simulink model "fll921"  (R2023a)
settings: Solver=ode45  StartTime=0.0  StopTime=0.12  RelTol=1e-6
model workspace (MAT data in the model file):
  K = 1
libraries: spsIGBTDiodeLib x6, spsabctoAlphaBetaZeroLib x4, spsAlphaBetaZerotoabcLib x2, spsAlphaBetaZerotodq0Lib x2, slpidlib x2, spsSawtoothGeneratorLib x2, cstextras x2, spsThreePhaseSeriesRLCBranchLib x2, spsThreePhaseVIMeasurementLib x2, spsGroundLib x1, spsDCVoltageSourceLib x1, spsSeriesRLCBranchLib x1
settings Model: Creator=Admin  LastModifiedBy=asus
settings SolverCC: ZeroCrossAlgorithm=Adaptive
settings DebuggingCC: IgnoredZcDiagnostic=none  UnconnectedInputMsg=warning  UnconnectedOutputMsg=warning  UnconnectedLineMsg=warning
settings ModelReferenceCC: EnableRefExpFcnMdlSchedulingChecks=on
settings RTWCC: DLArmComputeVersion=19.05

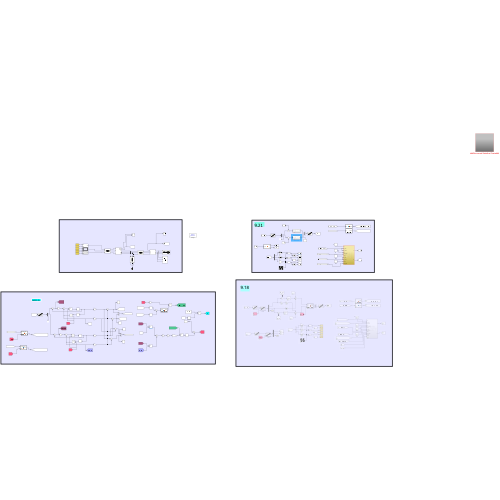
[thumbnail: Simulink's stored preview of the top-level diagram]
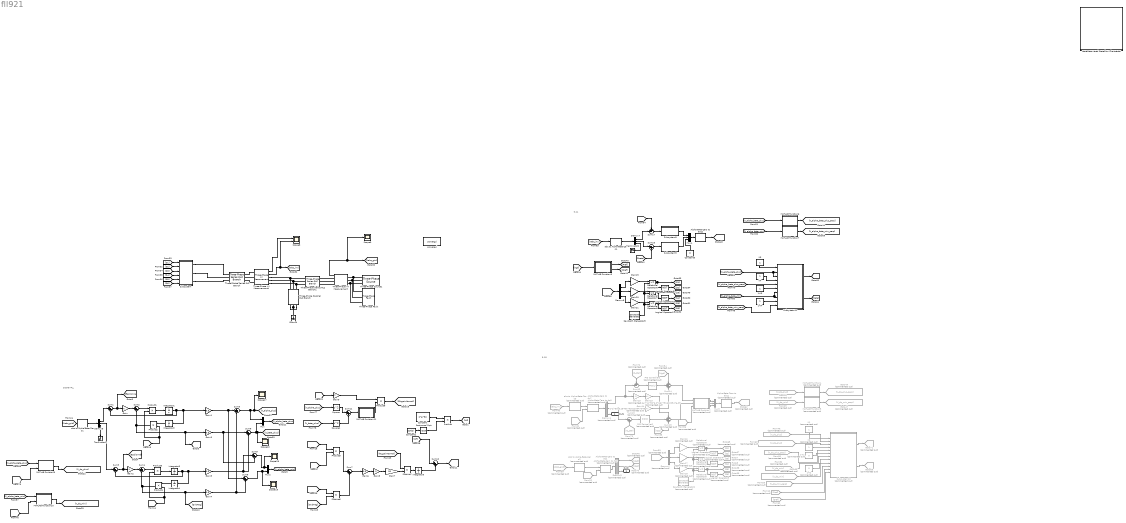
== system fll921 ==
  note: DSOGI-FLL
  note: 9.21
  note: 9.18
  ###Recovered Stateflow Charts### : Subsystem
  1-K1 : Constant  Commented=on  Value=0
  1-K2 : Constant  Commented=on  Value=0
  1-K3 : Constant
  1-K4 : Constant
  Alpha-Beta-Zero to abc1 : spsAlphaBetaZerotoabcLib/Alpha-Beta-Zero to abc  Commented=on
  Alpha-Beta-Zero to abc2 : spsAlphaBetaZerotoabcLib/Alpha-Beta-Zero to abc
  Alpha-Beta-Zero to dq1 : spsAlphaBetaZerotodq0Lib/Alpha-Beta-Zero to dq0  Commented=on  Alignment=90 degrees behind phase A axis
  Alpha-Beta-Zero to dq2 : spsAlphaBetaZerotodq0Lib/Alpha-Beta-Zero to dq0  Commented=on  Alignment=90 degrees behind phase A axis
  Constant : Constant  Value=2*pi*50
  Constant1 : Constant  Value=sqrt(2)
  Constant3 : Constant  Value=0
  Demux3 : Demux  Commented=on  Outputs=3
  Demux4 : Demux  Commented=on  Outputs=3
  Demux5 : Demux  Outputs=3
  Demux6 : Demux  Commented=on  Outputs=3
  Demux7 : Demux  Outputs=3
  Demux8 : Demux  Outputs=3
  From12 : From  Commented=on  GotoTag=Pref
  From20 : From  Commented=on  GotoTag=omega
  From21 : From  Commented=on  GotoTag=omega
  From28 : From  Commented=on  GotoTag=V_dq_plus
  From29 : From  Commented=on  GotoTag=V_dq_min
  From39 : From  Commented=on  GotoTag=Vabc_grid
  From40 : From  Commented=on  GotoTag=Iabc_inv
  From49 : From  Commented=on  GotoTag=V_dq_plus
  From50 : From  Commented=on  GotoTag=V_dq_plus_perp
  From52 : From  Commented=on  GotoTag=V_dq_min
  From53 : From  Commented=on  GotoTag=V_dq_min_perp
  From54 : From  Commented=on  GotoTag=Vgd
  From55 : From  Commented=on  GotoTag=Vgq
  From56 : From  Commented=on  GotoTag=omega
  From59 : From  Commented=on  GotoTag=Vabc_inv
  From62 : From  Commented=on  GotoTag=Qref
  From68 : From  Commented=on  GotoTag=V_dq_plus
  From69 : From  Commented=on  GotoTag=V_dq_min
  From72 : From  Commented=on  GotoTag=Id_star
  From73 : From  Commented=on  GotoTag=Iq_star
  Gain : Gain  Gain=K
  Gain{1,3..6} (5 alike) : Gain  Gain=0.5
  Gain13 : Gain  Commented=on  Gain=2*pi*50*6.254627916220947e-05
  Gain14 : Gain  Commented=on  Gain=2*pi*50*6.254627916220947e-05
  Gain15 : Gain  Commented=on  Gain=-1
  Gain16 : Gain  Commented=on  Gain=2/800
  Gain17 : Gain  Commented=on  Gain=2/800
  Gain18 : Gain  Commented=on  Gain=2/800
  Gain19 : Gain  Gain=2/800
  Gain2 : Gain  Gain=K
  Gain20 : Gain  Gain=2/800
  Gain21 : Gain  Gain=2/800
  Gain7 : Gain  Gain=50
  Gain8 : Gain  Gain=-1
  Gain9 : Gain  Gain=K
  Goto38 : Goto  Commented=on  GotoTag=S5
  Goto39 : Goto  Commented=on  GotoTag=S6
  Goto43 : Goto  Commented=on  GotoTag=V_dq_plus_perp
  Goto46 : Goto  Commented=on  GotoTag=Vgd
  Goto47 : Goto  Commented=on  GotoTag=V_dq_min_perp
  Goto62 : Goto  Commented=on  GotoTag=Vabc_inv
  Goto65 : Goto  Commented=on  GotoTag=S1
  Goto67 : Goto  Commented=on  GotoTag=S2
  Goto68 : Goto  Commented=on  GotoTag=Iq_star
  Goto7 : Goto  Commented=on  GotoTag=S3
  Goto70 : Goto  Commented=on  GotoTag=Vgq
  Goto71 : Goto  Commented=on  GotoTag=Id_star
  Goto8 : Goto  Commented=on  GotoTag=S4
  Ground : spsGroundLib/Ground  LConnTagsString=a
  Integrator{1..5} (5 alike) : Integrator
  "K1 " : Constant  Commented=on
  K2 : Constant  Commented=on
  K3 : Constant
  K4 : Constant
  Logical Operator10 : Logic  Operator=NOT  AllPortsSameDT=off  OutDataTypeStr=boolean
  Logical Operator11 : Logic  Operator=NOT  AllPortsSameDT=off  OutDataTypeStr=boolean
  Logical Operator3 : Logic  Commented=on  Operator=NOT  AllPortsSameDT=off  OutDataTypeStr=boolean
  Logical Operator4 : Logic  Commented=on  Operator=NOT  AllPortsSameDT=off  OutDataTypeStr=boolean
  Logical Operator5 : Logic  Commented=on  Operator=NOT  AllPortsSameDT=off  OutDataTypeStr=boolean
  Logical Operator9 : Logic  Operator=NOT  AllPortsSameDT=off  OutDataTypeStr=boolean
  MATLAB Function10 : MATLAB Function  TreatAsAtomicUnit=on
  MATLAB Function11 : MATLAB Function  TreatAsAtomicUnit=on
  MATLAB Function2 : MATLAB Function  Commented=on  TreatAsAtomicUnit=on
  MATLAB Function3 : MATLAB Function  TreatAsAtomicUnit=on
  MATLAB Function4 : MATLAB Function  Commented=on  TreatAsAtomicUnit=on
  MATLAB Function5 : MATLAB Function  Commented=on  TreatAsAtomicUnit=on
  MATLAB Function6 : MATLAB Function  TreatAsAtomicUnit=on
  MATLAB Function7 : MATLAB Function  TreatAsAtomicUnit=on
  MATLAB Function9 : MATLAB Function  TreatAsAtomicUnit=on
  Mux : Mux  Inputs=2
  Mux2 : Mux  Inputs=2
  Mux3 : Mux  Commented=on  Inputs=3
  Mux4 : Mux  Inputs=3
  PID Controller1 : slpidlib/PID Controller  Commented=on  Controller=PID  Form=Parallel  TimeDomain=Discrete-time  UseExternalTs=off  SampleTime=-1  IntegratorMethod=Forward Euler  FilterMethod=Forward Euler  ControllerParametersSource=internal  P=5  I=1  UseKiTs=off  D=0  N=100  UseFilter=on  TunerSelectOption=Transfer Function Based (PID Tuner App)  InitialConditionSource=internal  InitialConditionForIntegrator=0  InitialConditionForFilter=0  DifferentiatorICPrevScaledInput=0  ExternalReset=none  TrackingMode=off  Kt=1  LimitOutput=off  SatLimitsSource=internal  UpperSaturationLimit=inf  LowerSaturationLimit=-inf  LinearizeAsGain=on  AntiWindupMode=none  Kb=1  LimitIntegrator=off  UpperIntegratorSaturationLimit=inf  LowerIntegratorSaturationLimit=-inf  POutMin=[]  POutMax=[]  IOutMin=[]  IOutMax=[]  DOutMin=[]  DOutMax=[]  NOutMin=[]  NOutMax=[]  SumOutMin=[]  SumOutMax=[]  SaturationOutMin=[]  SaturationOutMax=[]  PParamMin=[]  PParamMax=[]  IParamMin=[]  IParamMax=[]  DParamMin=[]  DParamMax=[]  NParamMin=[]  NParamMax=[]  KbParamMin=[]  KbParamMax=[]  KtParamMin=[]  KtParamMax=[]  KbOutMin=[]  KbOutMax=[]  KtOutMin=[]  KtOutMax=[]  IntegratorOutMin=[]  IntegratorOutMax=[]  FilterOutMin=[]  FilterOutMax=[]  SumI1OutMin=[]  SumI1OutMax=[]  SumI2OutMin=[]  SumI2OutMax=[]  SumI3OutMin=[]  SumI3OutMax=[]  SumI4OutMin=[]  SumI4OutMax=[]  SumDOutMin=[]  SumDOutMax=[]  DifferentiatorOutMin=[]  DifferentiatorOutMax=[]  FilterDiffOutCoefMin=[]  FilterDiffOutCoefMax=[]  ReciprocalOutMin=[]  ReciprocalOutMax=[]  SumDenOutMin=[]  SumDenOutMax=[]  SumNumOutMin=[]  SumNumOutMax=[]  DivideOutMin=[]  DivideOutMax=[]  UdiffTsProdOutMin=[]  UdiffTsProdOutMax=[]  NTsProdOutMin=[]  NTsProdOutMax=[]  UintegralTsProdOutMin=[]  UintegralTsProdOutMax=[]  UngainTsProdOutMin=[]  UngainTsProdOutMax=[]  ClampingZeroOutDataTypeStr=Inherit: Inherit via back propagation  ClampingZeroOutMin=[]  ClampingZeroOutMax=[]  FilterDenConstantOutDataTypeStr=Inherit: Inherit via back propagation  FilterDenConstantOutMin=[]  FilterDenConstantOutMax=[]  PCopyOutDataTypeStr=Inherit: Inherit via back propagation  PCopyOutMin=[]  PCopyOutMax=[]  NCopyOutDataTypeStr=Inherit: Inherit via back propagation  NCopyOutMin=[]  NCopyOutMax=[]  IntegratorContinuousStateAttributes=''  IntegratorStateMustResolveToSignalObject=off  IntegratorRTWStateStorageClass=Auto  FilterContinuousStateAttributes=''  FilterStateMustResolveToSignalObject=off  FilterRTWStateStorageClass=Auto  ParallelPVariant=InternalParameters  IdealPVariant=Disabled  IVariant=InternalParameters  DVariant=InternalParameters  IntegratorVariant=Discrete  SatVariant=Disabled  AWVariant=Passthrough  PCopyVariant=Disabled  TRVariant=Disabled  FdbkBlocksVariant=Forward  IdealPFdbkVariant=Disabled  SatFdbkVariant=Disabled  DerivativeFilterVariant=ForwardEulerFilter  NVariant=InternalParameters  NCopyVariant=Disabled  FilterICVariant=InternalICsFilter  IntegratorICVariant=InternalICs  ExternalResetVariant=Disabled  TRSumVariant=Passthrough  SumFdbkVariant=Disabled  SumVariant=Sum_PID  TsampFilterVariant=InternalTs  TsampNgainVariant=Passthrough  TsampIntegralVariant=Disabled_SignalSpec  ExternalSaturationOutDataTypeStr=Inherit: Same as second input
  PID Controller2 : slpidlib/PID Controller  Commented=on  Controller=PID  Form=Parallel  TimeDomain=Discrete-time  UseExternalTs=off  SampleTime=-1  IntegratorMethod=Forward Euler  FilterMethod=Forward Euler  ControllerParametersSource=internal  P=5  I=1  UseKiTs=off  D=0  N=100  UseFilter=on  TunerSelectOption=Transfer Function Based (PID Tuner App)  InitialConditionSource=internal  InitialConditionForIntegrator=0  InitialConditionForFilter=0  DifferentiatorICPrevScaledInput=0  ExternalReset=none  TrackingMode=off  Kt=1  LimitOutput=off  SatLimitsSource=internal  UpperSaturationLimit=inf  LowerSaturationLimit=-inf  LinearizeAsGain=on  AntiWindupMode=none  Kb=1  LimitIntegrator=off  UpperIntegratorSaturationLimit=inf  LowerIntegratorSaturationLimit=-inf  POutMin=[]  POutMax=[]  IOutMin=[]  IOutMax=[]  DOutMin=[]  DOutMax=[]  NOutMin=[]  NOutMax=[]  SumOutMin=[]  SumOutMax=[]  SaturationOutMin=[]  SaturationOutMax=[]  PParamMin=[]  PParamMax=[]  IParamMin=[]  IParamMax=[]  DParamMin=[]  DParamMax=[]  NParamMin=[]  NParamMax=[]  KbParamMin=[]  KbParamMax=[]  KtParamMin=[]  KtParamMax=[]  KbOutMin=[]  KbOutMax=[]  KtOutMin=[]  KtOutMax=[]  IntegratorOutMin=[]  IntegratorOutMax=[]  FilterOutMin=[]  FilterOutMax=[]  SumI1OutMin=[]  SumI1OutMax=[]  SumI2OutMin=[]  SumI2OutMax=[]  SumI3OutMin=[]  SumI3OutMax=[]  SumI4OutMin=[]  SumI4OutMax=[]  SumDOutMin=[]  SumDOutMax=[]  DifferentiatorOutMin=[]  DifferentiatorOutMax=[]  FilterDiffOutCoefMin=[]  FilterDiffOutCoefMax=[]  ReciprocalOutMin=[]  ReciprocalOutMax=[]  SumDenOutMin=[]  SumDenOutMax=[]  SumNumOutMin=[]  SumNumOutMax=[]  DivideOutMin=[]  DivideOutMax=[]  UdiffTsProdOutMin=[]  UdiffTsProdOutMax=[]  NTsProdOutMin=[]  NTsProdOutMax=[]  UintegralTsProdOutMin=[]  UintegralTsProdOutMax=[]  UngainTsProdOutMin=[]  UngainTsProdOutMax=[]  ClampingZeroOutDataTypeStr=Inherit: Inherit via back propagation  ClampingZeroOutMin=[]  ClampingZeroOutMax=[]  FilterDenConstantOutDataTypeStr=Inherit: Inherit via back propagation  FilterDenConstantOutMin=[]  FilterDenConstantOutMax=[]  PCopyOutDataTypeStr=Inherit: Inherit via back propagation  PCopyOutMin=[]  PCopyOutMax=[]  NCopyOutDataTypeStr=Inherit: Inherit via back propagation  NCopyOutMin=[]  NCopyOutMax=[]  IntegratorContinuousStateAttributes=''  IntegratorStateMustResolveToSignalObject=off  IntegratorRTWStateStorageClass=Auto  FilterContinuousStateAttributes=''  FilterStateMustResolveToSignalObject=off  FilterRTWStateStorageClass=Auto  ParallelPVariant=InternalParameters  IdealPVariant=Disabled  IVariant=InternalParameters  DVariant=InternalParameters  IntegratorVariant=Discrete  SatVariant=Disabled  AWVariant=Passthrough  PCopyVariant=Disabled  TRVariant=Disabled  FdbkBlocksVariant=Forward  IdealPFdbkVariant=Disabled  SatFdbkVariant=Disabled  DerivativeFilterVariant=ForwardEulerFilter  NVariant=InternalParameters  NCopyVariant=Disabled  FilterICVariant=InternalICsFilter  IntegratorICVariant=InternalICs  ExternalResetVariant=Disabled  TRSumVariant=Passthrough  SumFdbkVariant=Disabled  SumVariant=Sum_PID  TsampFilterVariant=InternalTs  TsampNgainVariant=Passthrough  TsampIntegralVariant=Disabled_SignalSpec  ExternalSaturationOutDataTypeStr=Inherit: Same as second input
  Product{,1..8} (9 alike) : Product
  Reciprocal Sqrt : Sqrt  Operator=rSqrt  IntermediateResultsDataTypeStr=double
  Relational Operator3 : RelationalOperator  Commented=on  OutDataTypeStr=boolean  RndMeth=Simplest  InputSameDT=off
  Relational Operator4 : RelationalOperator  Commented=on  OutDataTypeStr=boolean  RndMeth=Simplest  InputSameDT=off
  Relational Operator5 : RelationalOperator  Commented=on  OutDataTypeStr=boolean  RndMeth=Simplest  InputSameDT=off
  Relational Operator6 : RelationalOperator  OutDataTypeStr=boolean  RndMeth=Simplest  InputSameDT=off
  Relational Operator7 : RelationalOperator  OutDataTypeStr=boolean  RndMeth=Simplest  InputSameDT=off
  Relational Operator8 : RelationalOperator  OutDataTypeStr=boolean  RndMeth=Simplest  InputSameDT=off
  Sawtooth Generator2 : spsSawtoothGeneratorLib/Sawtooth Generator  Commented=on  Freq=120e3  Phase=180  Ts=0
  Sawtooth Generator3 : spsSawtoothGeneratorLib/Sawtooth Generator  Freq=120e3  Phase=180  Ts=0
  Scope{9..10,17..19} (5 alike) : Scope
  Scope8 : Scope  NumInputPorts=2
  Square : Math  Operator=square
  Square1 : Math  Operator=square
  Subsystem : Subsystem
  Subsystem10 : Subsystem  Commented=on
  Subsystem11 : Subsystem
  Subsystem8 : Subsystem
  Subsystem9 : Subsystem
  Sum{1..5,9} (6 alike) : Sum  Inputs=|+-
  Sum{6..8,10..11} (5 alike) : Sum  Inputs=|++
  Sum12 : Sum  Commented=on  Inputs=+-|
  Sum13 : Sum  Commented=on  Inputs=|-+
  Sum14 : Sum  Commented=on  Inputs=+++
  Sum15 : Sum  Commented=on  Inputs=+++
  Sum16 : Sum  Inputs=|-+
  Sum17 : Sum  Inputs=+-|
  Terminator1 : Terminator
  Terminator2 : Terminator
  Three-Phase Parallel RLC Branch : spsThreePhaseParallelRLCBranchLib/Three-Phase Parallel RLC Branch  LConnTagsString=A|B|C  RConnTagsString=A|B|C  BranchType=C  Resistance=1  Inductance=1e-3  Capacitance=4.22171e-05  Measurements=None
  Three-Phase Series RLC Branch : spsThreePhaseSeriesRLCBranchLib/Three-Phase Series RLC Branch  LConnTagsString=A|B|C  RConnTagsString=A|B|C  BranchType=L  Resistance=1  Inductance=25.6e-06  Capacitance=1e-6  Measurements=None
  Three-Phase Series RLC Branch1 : spsThreePhaseSeriesRLCBranchLib/Three-Phase Series RLC Branch  LConnTagsString=A|B|C  RConnTagsString=A|B|C  BranchType=L  Resistance=1  Inductance=5e-06  Capacitance=1e-6  Measurements=None
  Three-Phase V-I Measurement : spsThreePhaseVIMeasurementLib/Three-Phase V-I Measurement  VoltageMeasurement=phase-to-ground  SetLabelV=off  LabelV=Vabc  Vpu=on  VpuLL=off  CurrentMeasurement=no  SetLabelI=off  LabelI=Iabc  Ipu=off  Pbase=100e6  Vbase=400  OutputType=Complex  PhasorSimulation=off  PSBequivalent=0
  Three-Phase V-I Measurement4 : spsThreePhaseVIMeasurementLib/Three-Phase V-I Measurement  VoltageMeasurement=phase-to-ground  SetLabelV=off  LabelV=Vabc  Vpu=on  VpuLL=off  CurrentMeasurement=yes  SetLabelI=off  LabelI=Iabc  Ipu=off  Pbase=100e6  Vbase=400  OutputType=Complex  PhasorSimulation=off  PSBequivalent=0
  Three-Phase Fault : spsThreePhaseFaultLib/Three-Phase Fault  InitialStates=0  FaultA=on  FaultB=on  FaultC=off  GroundFault=off  SwitchTimes="[0.08  0.1]"  External=off  SwitchStatus=NaN  FaultResistance=0.001  GroundResistance=0.01  SnubberResistance=1e6  SnubberCapacitance=inf  Measurements=Fault voltages
  Three-Phase Source1 : spsThreePhaseSourceLib/Three-Phase Source  InternalConnection=Yg  VoltagePhases=off  Voltage=400  PhaseAngle=0  Voltage_phases=[25e3 25e3 25e3]/sqrt(3)  PhaseAngles_phases=[0 -120 +120]  Frequency=50  NonIdealSource=on  SpecifyImpedance=off  Resistance=(3e-3*2*pi*50)/10  Inductance=3e-3  ShortCircuitLevel=160e3  BaseVoltage=400/sqrt(3)  XRratio=10  BusType=PQ  Pref=160e3  Qref=50000  Prefabc=[10e3, 10e3, 10e3]  Qrefabc=[0, 0, 0]  Qmin=-inf  Qmax=inf
  abc to Alpha-Beta-Zero1 : spsabctoAlphaBetaZeroLib/abc to Alpha-Beta-Zero
  abc to Alpha-Beta-Zero2 : spsabctoAlphaBetaZeroLib/abc to Alpha-Beta-Zero  Commented=on
  abc to Alpha-Beta-Zero3 : spsabctoAlphaBetaZeroLib/abc to Alpha-Beta-Zero  Commented=on
  abc to Alpha-Beta-Zero4 : spsabctoAlphaBetaZeroLib/abc to Alpha-Beta-Zero
  powergui : spspowerguiLib/powergui  Priority=1  SimulationMode=Discrete  SampleTime=6.024e-05  frequency=60  Iterations=50  frequencyindice=50  Pbase=100e6  ErrMax=1e-4  UnitsV=kV  UnitsW=MW  buscounter=0  FunctionMessages=off  echomessages=off  EnableUseOfTLC=off  CurrentSourceSwitches=off  DisableSnubberDevices=off  DisableRonSwitches=off  DisableVfSwitches=off  DisplayEquations=off  AutomaticDiscreteSolvers=off  SolverType=Tustin/Backward Euler (TBE)  Interpol=off  ExternalGateDelay=off  methode=off  Ts=100  x0status=blocks  SPID=on  SwTol=0  HookPort=off  NonlinearTolerance=1e-4  nMaxIteration=100  ContinueOnMaxIteration=off  RestoreLinks=warning  ResistiveCurrentMeasurement=off  Frange=[0:2:500]  Ylog=off  Xlog=on  ShowGrid=off  save=off  variable=ZData  structure=0  ZoomFFT=off  StartTime=0.0  cycles=1  DisplayStyle=1  fundamental=60  FreqAxis=off  MaxFrequency=1000  frequencyindicesteady=1  RmsSteady=1  display=off
  Out1 : Outport
  Out2 : Outport  Port=2
  wires:
  Reciprocal Sqrt/1 -> Product/2
  Constant/1 -> Product/1
  Constant1/1 -> Reciprocal Sqrt/1
  Product/1 -> [Wf]
  abc to Alpha-Beta-Zero1/1 -> Demux5/1
  Demux5/1 -> Sum1/1
  Sum1/1 -> [EpsilonVa], Gain/1
  Gain/1 -> Sum2/1
  Sum2/1 -> Product1/1
  Product1/1 -> Integrator1/1
  Integrator1/1 -> Sum1/2, Gain1/1, Integrator2/1
  Integrator2/1 -> Product2/1
  [omega] -> Product2/2, Product1/2
  Product2/1 -> [QvaTag], Gain3/1, Sum2/2
  Sum4/1 -> Product3/1
  Gain2/1 -> Sum4/1
  Integrator3/1 -> Sum3/2, Gain5/1, Integrator4/1
  Product3/1 -> Integrator3/1
  [omega] -> Product4/2, Product3/2
  Integrator4/1 -> Product4/1
  Demux5/2 -> Sum3/1
  Sum3/1 -> [EpsilonVb], Gain2/1
  Gain1/1 -> Sum5/1, Sum6/1
  Gain4/1 -> Sum6/2, Sum5/2
  Sum5/1 -> Mux/1, Scope17/1, [V_alpha_plus]
  Sum6/1 -> Scope19/1, Mux2/2
  Gain3/1 -> Sum8/1, Sum9/2
  Gain5/1 -> Sum9/1, Sum8/2
  Sum8/1 -> Scope10/1, [V_beta_plus], Mux/2
  Sum9/1 -> Scope18/1, Mux2/1
  Product4/1 -> Gain4/1, [QvbTag], Sum4/2
  [EpsilonVa] -> Product5/1
  [QvaTag] -> Product5/2
  [EpsilonVb] -> Product6/1
  [QvbTag] -> Product6/2
  Product5/1 -> Sum7/1
  Product6/1 -> Sum7/2
  Sum7/1 -> Gain6/1
  Gain6/1 -> Gain8/1
  Gain8/1 -> Gain7/1
  Integrator5/1 -> Sum10/2
  [Wf] -> Sum10/1
  Sum10/1 -> [omega]
  [V_alpha_plus] -> Square/1
  [V_beta_plus] -> Square1/1
  Square1/1 -> Sum11/2
  Square/1 -> Sum11/1
  [omega] -> Gain9/1
  Gain9/1 -> Product8/1
  Product8/1 -> [FLLgainNormal]
  [FLLgainNormal] -> Product7/1
  [Vabc_grid] -> abc to Alpha-Beta-Zero1/1
  Three-Phase V-I Measurement4/2 -> Scope8/2, [Iabc_inv]
  [S5] -> Subsystem/5(S5)
  [S1] -> Subsystem/1(S1)
  [S4] -> Subsystem/4(S4)
  [S3] -> Subsystem/3(S3)
  [S2] -> Subsystem/2(S2)
  [S6] -> Subsystem/6(S6)
  Three-Phase V-I Measurement4/1 -> Scope8/1
  Three-Phase V-I Measurement/1 -> Scope9/1, [Vabc_grid]
  Subsystem11/1(Out1) -> [Ialpha]
  [V_alpha_beta_plus] -> Subsystem11/3(V_plus1), Subsystem11/2(V_plus)
  K4/1 -> Subsystem11/4(K2)
  [V_alpha_beta_plus_perp] -> Subsystem11/5(plus_perp)
  1-K3/1 -> Subsystem11/6(1-K1)
  K3/1 -> Subsystem11/1(K1)
  Gain19/1 -> Relational Operator6/1
  [V_alpha_beta_min] -> Subsystem11/7(V_min), Subsystem11/8(V_min1)
  Demux7/2 -> Sum16/1
  1-K4/1 -> Subsystem11/9(1-K2)
  Relational Operator7/1 -> Logical Operator10/1, [S3]
  Subsystem9/1(Out1) -> Mux4/2
  Subsystem10/2(Out2) -> Goto68/1
  Subsystem10/1(Out1) -> Goto71/1
  Gain13/1 -> Sum15/1
  Demux3/2 -> Goto70/1
  From52/1 -> Subsystem10/7(V_min)
  Demux6/2 -> Gain17/1
  1-K2/1 -> Subsystem10/9(1-K2)
  From49/1 -> Subsystem10/2(V_plus)
  From39/1 -> abc to Alpha-Beta-Zero2/1
  Logical Operator4/1 -> Goto8/1
  "K1 "/1 -> Subsystem10/1(K1)
  1-K1/1 -> Subsystem10/6(1-K1)
  Demux7/1 -> Sum17/2
  Gain14/1 -> Sum14/3
  Sum17/1 -> Subsystem8/1(In1)
  Logical Operator10/1 -> [S4]
  MATLAB Function4/1(V_perp) -> Goto43/1
  K2/1 -> Subsystem10/4(K2)
  Sum12/1 -> PID Controller1/1
  From68/1 -> Subsystem10/3(V_plus1)
  Subsystem11/2(Out2) -> [Ibeta]
  abc to Alpha-Beta-Zero4/1 -> Demux7/1
  Logical Operator3/1 -> Goto67/1
  Subsystem8/1(Out1) -> Mux4/1
  Demux8/1 -> Gain19/1
  From59/1 -> Demux6/1
  [Vabc_inv] -> Demux8/1
  Sawtooth Generator3/1 -> Relational Operator6/2, Relational Operator7/2, Relational Operator8/2
  Gain17/1 -> Relational Operator4/1
  Logical Operator9/1 -> [S2]
  Sum16/1 -> Subsystem9/1(In1)
  From53/1 -> Subsystem10/10(min_perp)
  Relational Operator3/1 -> Goto65/1, Logical Operator3/1
  [Ibeta] -> Sum16/2
  MATLAB Function5/1(V_perp) -> Goto47/1
  From56/1 -> MATLAB Function2/3(theta)
  Logical Operator11/1 -> [S6]
  Alpha-Beta-Zero to dq2/1 -> Demux4/1
  Gain15/1 -> Gain13/1
  Demux8/3 -> Gain21/1
  Relational Operator8/1 -> [S5], Logical Operator11/1
  Mux4/1 -> Alpha-Beta-Zero to abc2/1
  Gain20/1 -> Relational Operator7/1
  Logical Operator5/1 -> Goto39/1
  [Iabc_inv] -> abc to Alpha-Beta-Zero4/1
  From72/1 -> Sum12/1
  From54/1 -> Sum14/1
  PID Controller1/1 -> Sum14/2
  From40/1 -> abc to Alpha-Beta-Zero3/1
  Sum13/1 -> PID Controller2/1
  Alpha-Beta-Zero to dq1/1 -> Demux3/1
  Mux3/1 -> Alpha-Beta-Zero to abc1/1
  Demux4/3 -> Out1/1
  Alpha-Beta-Zero to abc2/1 -> [Vabc_inv]
  Gain18/1 -> Relational Operator5/1
  abc to Alpha-Beta-Zero2/1 -> Alpha-Beta-Zero to dq1/1
  Demux4/2 -> Sum13/1, Gain14/1
  From20/1 -> Alpha-Beta-Zero to dq1/2
  From21/1 -> Alpha-Beta-Zero to dq2/2
  Demux6/3 -> Gain18/1
  Relational Operator4/1 -> Logical Operator4/1, Goto7/1
  Demux3/1 -> Goto46/1
  Alpha-Beta-Zero to abc1/1 -> Goto62/1
  abc to Alpha-Beta-Zero3/1 -> Alpha-Beta-Zero to dq2/1
  PID Controller2/1 -> Sum15/2
  Gain16/1 -> Relational Operator3/1
  MATLAB Function6/1(V_perp) -> [V_alpha_beta_plus_perp]
  [Ialpha] -> Sum17/1
  From50/1 -> Subsystem10/5(plus_perp)
  MATLAB Function7/1(V_perp) -> [V_alpha_beta_min_perp]
  Demux3/3 -> Out2/1
  From55/1 -> Sum15/3
  Demux4/1 -> Gain15/1, Sum12/2
  Relational Operator6/1 -> [S1], Logical Operator9/1
  Sawtooth Generator2/1 -> Relational Operator3/2, Relational Operator4/2, Relational Operator5/2
  Relational Operator5/1 -> Goto38/1, Logical Operator5/1
  Gain21/1 -> Relational Operator8/1
  [V_alpha_beta_min_perp] -> Subsystem11/10(min_perp)
  Demux8/2 -> Gain20/1
  Demux6/1 -> Gain16/1
  From73/1 -> Sum13/2
  From69/1 -> Subsystem10/8(V_min1)
  Mux/1 -> [V_alpha_beta_plus]
  Mux2/1 -> [V_alpha_beta_min]
  From29/1 -> MATLAB Function5/1(V)
  From28/1 -> MATLAB Function4/1(V)
  [V_alpha_beta_plus] -> MATLAB Function6/1(V)
  [V_alpha_beta_min] -> MATLAB Function7/1(V)
  From12/1 -> Subsystem10/11(Pref)
  From62/1 -> Subsystem10/12(Qref1)
  MATLAB Function2/2(V_beta) -> Mux3/2
  MATLAB Function2/1(V_alpha) -> Mux3/1
  MATLAB Function2/3(V_zero) -> Mux3/3
  Sum15/1 -> MATLAB Function2/2(V_q)
  Sum14/1 -> MATLAB Function2/1(V_d)
  [omega] -> MATLAB Function9/2(theta)
  [V_alpha_beta_plus] -> MATLAB Function9/1(V_alpha_beta)
  MATLAB Function9/1(V_dq) -> [V_dq_plus]
  [V_alpha_beta_min] -> MATLAB Function10/1(V_alpha_beta)
  [omega] -> MATLAB Function10/2(theta)
  MATLAB Function10/1(V_dq) -> [V_dq_min]
  Demux5/3 -> Terminator1/1
  Gain7/1 -> Product7/2
  Product7/1 -> Integrator5/1
  Sum11/1 -> MATLAB Function11/1(input)
  MATLAB Function11/1(result) -> Product8/2
  Demux7/3 -> Terminator2/1
  Constant3/1 -> Mux4/3
  [Vgd] -> MATLAB Function3/1(V_pu)
  MATLAB Function3/1(P) -> [Pref]
  MATLAB Function3/2(Q) -> [Qref]
  connections:
  Three-Phase Parallel RLC Branch/RConn2 -- Ground/LConn1 -- Three-Phase Parallel RLC Branch/RConn3 -- Three-Phase Parallel RLC Branch/RConn1
  Three-Phase V-I Measurement4/RConn2 -- Three-Phase Series RLC Branch1/LConn2 -- Three-Phase Parallel RLC Branch/LConn2
  Three-Phase V-I Measurement4/RConn1 -- Three-Phase Series RLC Branch1/LConn1 -- Three-Phase Parallel RLC Branch/LConn1
  Three-Phase V-I Measurement4/RConn3 -- Three-Phase Series RLC Branch1/LConn3 -- Three-Phase Parallel RLC Branch/LConn3
  Subsystem/RConn2 -- Three-Phase Series RLC Branch/LConn2
  Subsystem/RConn3 -- Three-Phase Series RLC Branch/LConn3
  Three-Phase V-I Measurement4/LConn1 -- Three-Phase Series RLC Branch/RConn1
  Three-Phase V-I Measurement4/LConn3 -- Three-Phase Series RLC Branch/RConn3
  Three-Phase V-I Measurement4/LConn2 -- Three-Phase Series RLC Branch/RConn2
  Subsystem/RConn1 -- Three-Phase Series RLC Branch/LConn1
  Three-Phase Source1/RConn1 -- Three-Phase Fault/LConn1 -- Three-Phase V-I Measurement/LConn1
  Three-Phase Source1/RConn2 -- Three-Phase Fault/LConn2 -- Three-Phase V-I Measurement/LConn2
  Three-Phase Source1/RConn3 -- Three-Phase Fault/LConn3 -- Three-Phase V-I Measurement/LConn3
  Three-Phase V-I Measurement/RConn1 -- Three-Phase Series RLC Branch1/RConn1
  Three-Phase V-I Measurement/RConn2 -- Three-Phase Series RLC Branch1/RConn2
  Three-Phase V-I Measurement/RConn3 -- Three-Phase Series RLC Branch1/RConn3

== system fll921/###Recovered Stateflow Charts### ==

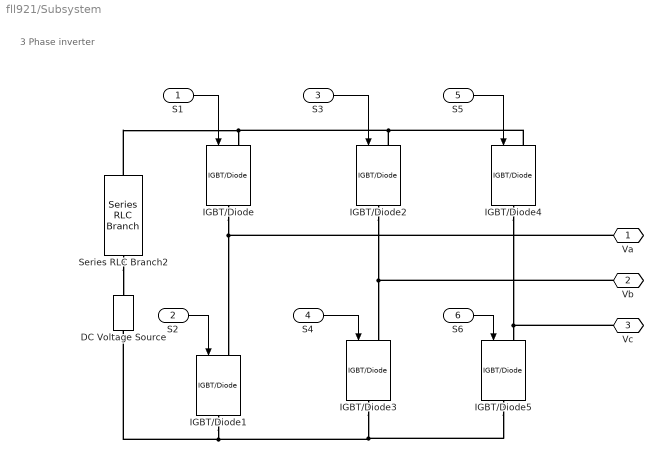
== system fll921/Subsystem ==
  note: 3 Phase inverter
  S1 : Inport
  S2 : Inport  Port=2
  S3 : Inport  Port=3
  S4 : Inport  Port=4
  S5 : Inport  Port=5
  S6 : Inport  Port=6
  DC Voltage Source : spsDCVoltageSourceLib/DC Voltage Source  Amplitude=800  Measurements=None
  IGBT/Diode{,1..5} (6 alike) : spsIGBTDiodeLib/IGBT//Diode  Ron=0.01  Rs=10  Cs=0.1e-6  Measurements=off
  Series RLC Branch2 : spsSeriesRLCBranchLib/Series RLC Branch  LConnTagsString=__new0  RConnTagsString=__new0  BranchType=R  Resistance=0.01  Inductance=1e-3  SetiL0=off  InitialCurrent=0  Capacitance=1e-6  Setx0=off  InitialVoltage=0  Measurements=None
  Va : PMIOPort  Side=Right
  Vb : PMIOPort  Port=2  Side=Right
  Vc : PMIOPort  Port=3  Side=Right
  wires:
  S1/1 -> IGBT/Diode/1
  S2/1 -> IGBT/Diode1/1
  S4/1 -> IGBT/Diode3/1
  S5/1 -> IGBT/Diode4/1
  S3/1 -> IGBT/Diode2/1
  S6/1 -> IGBT/Diode5/1
  connections:
  IGBT/Diode2/RConn1 -- Vb/RConn1 -- IGBT/Diode3/LConn1
  IGBT/Diode/RConn1 -- Va/RConn1 -- IGBT/Diode1/LConn1
  IGBT/Diode2/LConn1 -- Series RLC Branch2/RConn1 -- IGBT/Diode/LConn1 -- IGBT/Diode4/LConn1
  IGBT/Diode3/RConn1 -- IGBT/Diode1/RConn1 -- DC Voltage Source/LConn1 -- IGBT/Diode5/RConn1
  IGBT/Diode4/RConn1 -- Vc/RConn1 -- IGBT/Diode5/LConn1
  Series RLC Branch2/LConn1 -- DC Voltage Source/RConn1

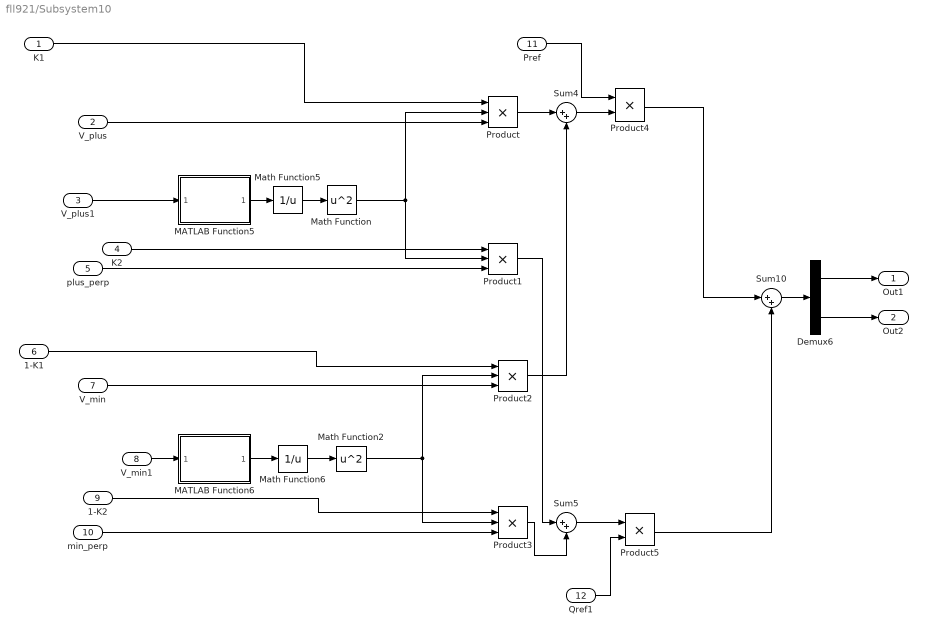
== system fll921/Subsystem10 ==
  K1 : Inport
  V_plus : Inport  Port=2
  V_plus1 : Inport  Port=3
  K2 : Inport  Port=4
  plus_perp : Inport  Port=5
  1-K1 : Inport  Port=6
  V_min : Inport  Port=7
  V_min1 : Inport  Port=8
  1-K2 : Inport  Port=9
  min_perp : Inport  Port=10
  Pref : Inport  Port=11
  Qref1 : Inport  Port=12
  Demux6 : Demux  Outputs=2
  MATLAB Function5 : MATLAB Function  TreatAsAtomicUnit=on
  MATLAB Function6 : MATLAB Function  TreatAsAtomicUnit=on
  Math Function : Math  Operator=square
  Math Function2 : Math  Operator=square
  Math Function5 : Math  Operator=reciprocal
  Math Function6 : Math  Operator=reciprocal
  Product{,1..3} (4 alike) : Product  Inputs=3
  Product4 : Product
  Product5 : Product
  Sum10 : Sum  Inputs=|++
  Sum4 : Sum  Inputs=|++
  Sum5 : Sum  Inputs=|++
  Out1 : Outport
  Out2 : Outport  Port=2
  wires:
  MATLAB Function5/1(v_norm_squared) -> Math Function5/1
  Product3/1 -> Sum5/2
  Math Function6/1 -> Math Function2/1
  Math Function2/1 -> Product2/2, Product3/2
  min_perp/1 -> Product3/3
  Math Function/1 -> Product1/2, Product/2
  Sum5/1 -> Product5/1
  Sum4/1 -> Product4/2
  Product/1 -> Sum4/1
  Product5/1 -> Sum10/2
  K2/1 -> Product1/1
  Demux6/2 -> Out2/1
  1-K1/1 -> Product2/1
  Product4/1 -> Sum10/1
  MATLAB Function6/1(v_norm_squared) -> Math Function6/1
  V_min/1 -> Product2/3
  Product1/1 -> Sum5/1
  Math Function5/1 -> Math Function/1
  Product2/1 -> Sum4/2
  V_min1/1 -> MATLAB Function6/1(V_alpha_beta)
  V_plus1/1 -> MATLAB Function5/1(V_alpha_beta)
  Sum10/1 -> Demux6/1
  Qref1/1 -> Product5/2
  V_plus/1 -> Product/3
  plus_perp/1 -> Product1/3
  1-K2/1 -> Product3/1
  K1/1 -> Product/1
  Demux6/1 -> Out1/1
  Pref/1 -> Product4/1

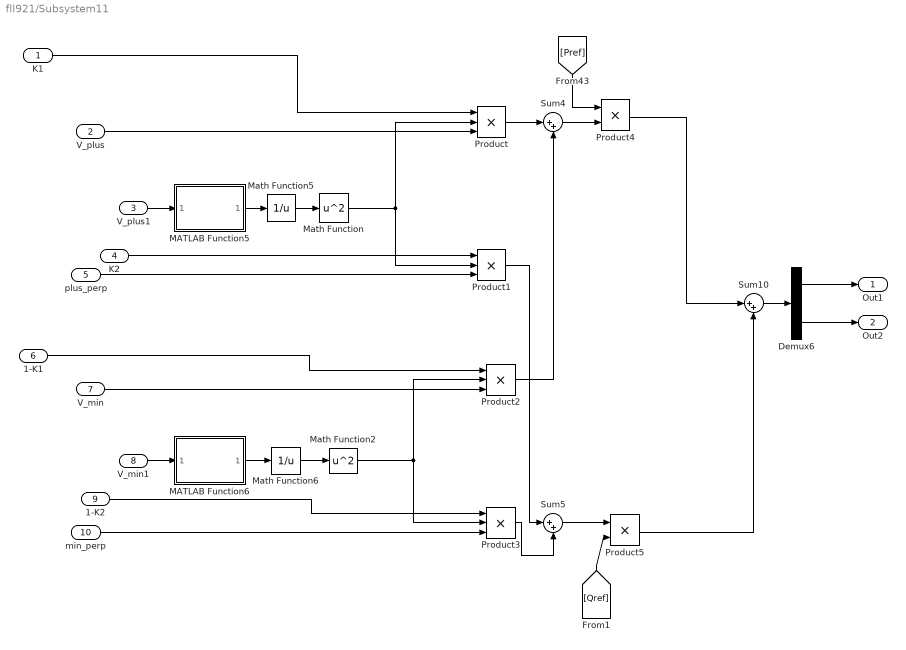
== system fll921/Subsystem11 ==
  K1 : Inport
  V_plus : Inport  Port=2
  V_plus1 : Inport  Port=3
  K2 : Inport  Port=4
  plus_perp : Inport  Port=5
  1-K1 : Inport  Port=6
  V_min : Inport  Port=7
  V_min1 : Inport  Port=8
  1-K2 : Inport  Port=9
  min_perp : Inport  Port=10
  Demux6 : Demux  Outputs=2
  MATLAB Function5 : MATLAB Function  TreatAsAtomicUnit=on
  MATLAB Function6 : MATLAB Function  TreatAsAtomicUnit=on
  Math Function : Math  Operator=square
  Math Function2 : Math  Operator=square
  Math Function5 : Math  Operator=reciprocal
  Math Function6 : Math  Operator=reciprocal
  Product{,1..3} (4 alike) : Product  Inputs=3
  Product4 : Product
  Product5 : Product
  Sum10 : Sum  Inputs=|++
  Sum4 : Sum  Inputs=|++
  Sum5 : Sum  Inputs=|++
  Out1 : Outport
  Out2 : Outport  Port=2
  wires:
  MATLAB Function5/1(v_norm_squared) -> Math Function5/1
  Product3/1 -> Sum5/2
  Math Function6/1 -> Math Function2/1
  Math Function2/1 -> Product2/2, Product3/2
  min_perp/1 -> Product3/3
  Math Function/1 -> Product1/2, Product/2
  Sum5/1 -> Product5/1
  Sum4/1 -> Product4/2
  Product/1 -> Sum4/1
  Product5/1 -> Sum10/2
  K2/1 -> Product1/1
  Demux6/2 -> Out2/1
  1-K1/1 -> Product2/1
  Product4/1 -> Sum10/1
  MATLAB Function6/1(v_norm_squared) -> Math Function6/1
  V_min/1 -> Product2/3
  Product1/1 -> Sum5/1
  Math Function5/1 -> Math Function/1
  Product2/1 -> Sum4/2
  V_min1/1 -> MATLAB Function6/1(V_alpha_beta)
  V_plus1/1 -> MATLAB Function5/1(V_alpha_beta)
  Sum10/1 -> Demux6/1
  [Qref] -> Product5/2
  [Pref] -> Product4/1
  V_plus/1 -> Product/3
  plus_perp/1 -> Product1/3
  1-K2/1 -> Product3/1
  K1/1 -> Product/1
  Demux6/1 -> Out1/1

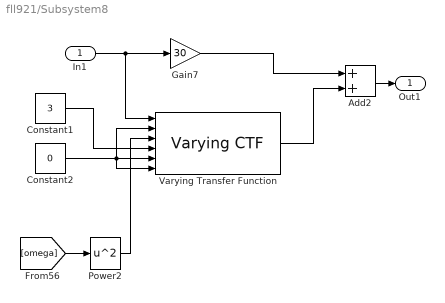
== system fll921/Subsystem8 ==
  In1 : Inport
  Add2 : Sum
  Constant1 : Constant  Value=3
  Constant2 : Constant  Value=0
  Gain7 : Gain  Gain=30
  Power2 : Math  Operator=square
  Varying Transfer Function : cstextras/Varying CTF  N=2
  Out1 : Outport
  wires:
  In1/1 -> Varying Transfer Function/1, Gain7/1
  Gain7/1 -> Add2/1
  Constant1/1 -> Varying Transfer Function/4
  Varying Transfer Function/1 -> Add2/2
  Add2/1 -> Out1/1
  [omega] -> Power2/1
  Constant2/1 -> Varying Transfer Function/2, Varying Transfer Function/6, Varying Transfer Function/5
  Power2/1 -> Varying Transfer Function/3

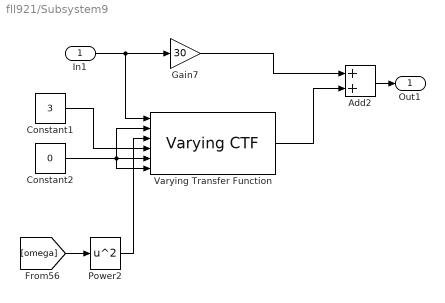
== system fll921/Subsystem9 ==
  In1 : Inport
  Add2 : Sum
  Constant1 : Constant  Value=3
  Constant2 : Constant  Value=0
  Gain7 : Gain  Gain=30
  Power2 : Math  Operator=square
  Varying Transfer Function : cstextras/Varying CTF  N=2
  Out1 : Outport
  wires:
  In1/1 -> Varying Transfer Function/1, Gain7/1
  Gain7/1 -> Add2/1
  Constant1/1 -> Varying Transfer Function/4
  Varying Transfer Function/1 -> Add2/2
  Add2/1 -> Out1/1
  Power2/1 -> Varying Transfer Function/3
  [omega] -> Power2/1
  Constant2/1 -> Varying Transfer Function/5, Varying Transfer Function/6, Varying Transfer Function/2

== matlab function fll921/Subsystem10/MATLAB Function6 ==
  data: V_alpha_beta input; v_norm_squared output
function v_norm_squared = calculateNormSquared(V_alpha_beta)
    v_norm_squared = V_alpha_beta(1)^2 + V_alpha_beta(2)^2;
    if v_norm_squared == 0
        v_norm_squared = NaN;
    end
end

== matlab function fll921/MATLAB Function2 ==
  data: V_d input; V_alpha output; V_q input; theta input; V_beta output; V_zero output
function [V_alpha, V_beta, V_zero] = dq_to_alpha_beta_zero(V_d, V_q, theta)
    % dq_to_alpha_beta_zero: Converts V_d, V_q to V_alpha, V_beta, and V_zero
    %
    % Inputs:
    %   V_d    - Direct-axis voltage component
    %   V_q    - Quadrature-axis voltage component
    %   theta  - Angle of the rotating frame (in radians)
    %
    % Outputs:
    %   V_alpha - Alpha-axis (stationary) voltage component
    %   V_beta  - Beta-axis (stationary) voltage component
    %   V_zero  - Zero-sequence voltage component (typically zero for balanced systems)

    % Compute V_alpha and V_beta using the inverse Park transformation
    V_alpha = V_d * cos(theta) - V_q * sin(theta);
    V_beta  = V_d * sin(theta) + V_q * cos(theta);

    % Compute V_zero (zero-sequence component)
    V_zero = 0;  % Set to zero if there's no zero-sequence component in the system
end

== matlab function fll921/Subsystem11/MATLAB Function5 ==
  data: V_alpha_beta input; v_norm_squared output
function v_norm_squared = calculateNormSquared(V_alpha_beta)
    v_norm_squared = V_alpha_beta(1)^2 + V_alpha_beta(2)^2;
end

== matlab function fll921/Subsystem11/MATLAB Function6 ==
  data: V_alpha_beta input; v_norm_squared output
function v_norm_squared = calculateNormSquared(V_alpha_beta)
    v_norm_squared = V_alpha_beta(1)^2 + V_alpha_beta(2)^2;
end

== matlab function fll921/MATLAB Function9 ==
  data: V_alpha_beta input; V_dq output; theta input
function V_dq = alphaBetaToDQ(V_alpha_beta, theta)
    % V_alpha_beta הוא וקטור דו-ממדי בגודל 2 המכיל את רכיבי האלפא-בטא
    % theta היא הזווית להמרה לתצורת d-q
    
    % חלץ את רכיבי האלפא והבטא
    V_alpha = V_alpha_beta(1);
    V_beta = V_alpha_beta(2);
    
    % בצע את טרנספורמציית ה-Park לתצורת d-q
    V_d = V_alpha * cos(theta) + V_beta * sin(theta);
    V_q = -V_alpha * sin(theta) + V_beta * cos(theta);
    
    % החזר את הווקטור d-q בגודל 2
    V_dq = [V_d; V_q];
end

== matlab function fll921/MATLAB Function10 ==
  data: V_alpha_beta input; V_dq output; theta input
function V_dq = alphaBetaToDQ(V_alpha_beta, theta)
    % V_alpha_beta הוא וקטור דו-ממדי בגודל 2 המכיל את רכיבי האלפא-בטא
    % theta היא הזווית להמרה לתצורת d-q
    
    % חלץ את רכיבי האלפא והבטא
    V_alpha = V_alpha_beta(1);
    V_beta = V_alpha_beta(2);
    
    % בצע את טרנספורמציית ה-Park לתצורת d-q
    V_d = V_alpha * cos(theta) + V_beta * sin(theta);
    V_q = -V_alpha * sin(theta) + V_beta * cos(theta);
    
    % החזר את הווקטור d-q בגודל 2
    V_dq = [V_d; V_q];
end

== matlab function fll921/MATLAB Function11 ==
  data: input input; result output
function result = safeReciprocal(input)
    % Define a small epsilon to avoid division by zero
    epsilon = 1e-6;

    % Calculate the reciprocal, adding epsilon if input is zero or very small
    if abs(input) < epsilon
        result = 1 / epsilon; % or any default value you prefer
    else
        result = 1 / input;
    end
end

== matlab function fll921/MATLAB Function3 ==
  data: V_pu input; P output; Q output
function [P, Q] = PowerControlLogic(V_pu)
       % Constants
       V_high_threshold = 0.85;  % Upper voltage threshold
       V_low_threshold = 0.4;   % Lower voltage threshold
       S_total = 160;            % Total apparent power (kVA)
       
       % Power Injection Logic
       if V_pu >= V_high_threshold
           % Only active power
           P = S_total;
           Q = 0;
       elseif V_pu <= V_low_threshold
           % Only reactive power
           P = 0;
           Q = S_total;
       else
           % Linear interpolation between thresholds
           power_ratio = (V_high_threshold - V_pu) / ...
                         (V_high_threshold - V_low_threshold);
           
           P = S_total * (1 - power_ratio);
           Q = S_total * power_ratio;
       end
   end

== matlab function fll921/MATLAB Function4 ==
  data: V input; V_perp output
function V_perp = calculatePerpendicular(V)
    % V הוא וקטור דו-ממדי עם שני רכיבים, למשל [V_alpha; V_beta] או [V_d; V_q]
    V1 = V(1);  % הרכיב הראשון של הווקטור (למשל V_alpha או V_d)
    V2 = V(2);  % הרכיב השני של הווקטור (למשל V_beta או V_q)
    
    % חישוב הרכיב הניצב
    V_perp = [-V2; V1];
end

== matlab function fll921/MATLAB Function5 ==
  data: V input; V_perp output
function V_perp = calculatePerpendicular(V)
    % V הוא וקטור דו-ממדי עם שני רכיבים, למשל [V_alpha; V_beta] או [V_d; V_q]
    V1 = V(1);  % הרכיב הראשון של הווקטור (למשל V_alpha או V_d)
    V2 = V(2);  % הרכיב השני של הווקטור (למשל V_beta או V_q)
    
    % חישוב הרכיב הניצב
    V_perp = [-V2; V1];
end

== matlab function fll921/MATLAB Function6 ==
  data: V input; V_perp output
function V_perp = calculatePerpendicular(V)
    % V הוא וקטור דו-ממדי עם שני רכיבים, למשל [V_alpha; V_beta] או [V_d; V_q]
    V1 = V(1);  % הרכיב הראשון של הווקטור (למשל V_alpha או V_d)
    V2 = V(2);  % הרכיב השני של הווקטור (למשל V_beta או V_q)
    
    % חישוב הרכיב הניצב
    V_perp = [-V2; V1];
end

== matlab function fll921/MATLAB Function7 ==
  data: V input; V_perp output
function V_perp = calculatePerpendicular(V)
    % V הוא וקטור דו-ממדי עם שני רכיבים, למשל [V_alpha; V_beta] או [V_d; V_q]
    V1 = V(1);  % הרכיב הראשון של הווקטור (למשל V_alpha או V_d)
    V2 = V(2);  % הרכיב השני של הווקטור (למשל V_beta או V_q)
    
    % חישוב הרכיב הניצב
    V_perp = [-V2; V1];
end

== matlab function fll921/Subsystem10/MATLAB Function5 ==
  data: V_alpha_beta input; v_norm_squared output
function v_norm_squared = calculateNormSquared(V_alpha_beta)
    v_norm_squared = V_alpha_beta(1)^2 + V_alpha_beta(2)^2;
    if v_norm_squared == 0
        v_norm_squared = NaN;
    end
end
